simulink model "Khan_hw_3"  (R2021a)
settings: Solver=VariableStepAuto  StartTime=0.0  StopTime=10.0  RelTol=1e-3
values from neighbouring files (symbols this model uses):
  q0 = angle2quat(phidot,thetadot,psidot)    [khan_hw_3_script.m]
settings Model: Creator=ARK  LastModifiedBy=ARK

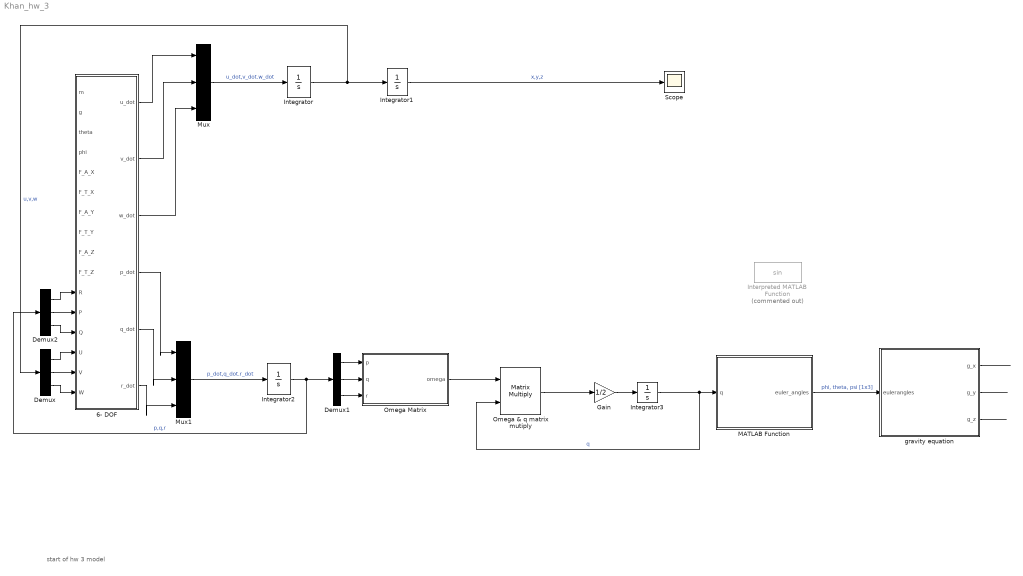
== system Khan_hw_3 ==
  note: start of hw 3 model
  6- DOF : MATLAB Function  TreatAsAtomicUnit=on
  Demux : Demux  Outputs=3
  Demux1 : Demux  Outputs=3
  Demux2 : Demux  Outputs=3
  Gain : Gain  Gain=1/2
  Integrator : Integrator  InitialCondition=1
  Integrator1 : Integrator  InitialCondition=1
  Integrator2 : Integrator  InitialCondition=1
  Integrator3 : Integrator  InitialCondition=q0
  Interpreted MATLAB Function : MATLABFcn  Commented=on
  MATLAB Function : MATLAB Function  TreatAsAtomicUnit=on
  Mux : Mux  Inputs=3
  Mux1 : Mux  Inputs=3
  Omega & q matrix mutiply : Product  Multiplication=Matrix(*)
  Omega Matrix : MATLAB Function  TreatAsAtomicUnit=on
  Scope : Scope
  gravity equation : MATLAB Function  TreatAsAtomicUnit=on
  wires:
  6- DOF/1(u_dot) -> Mux/1
  6- DOF/2(v_dot) -> Mux/2
  6- DOF/3(w_dot) -> Mux/3
  Mux/1 -> Integrator/1  "u_dot,v_dot.w_dot"
  Integrator/1 -> Integrator1/1, Demux/1  "u,v,w"
  Integrator1/1 -> Scope/1  "x,y,z"
  Demux/2 -> 6- DOF/15(V)
  Demux/1 -> 6- DOF/14(U)
  Demux/3 -> 6- DOF/16(W)
  6- DOF/4(p_dot) -> Mux1/1
  6- DOF/5(q_dot) -> Mux1/2
  6- DOF/6(r_dot) -> Mux1/3
  Mux1/1 -> Integrator2/1  "p_dot,q_dot.r_dot"
  Integrator2/1 -> Demux2/1, Demux1/1  "p,q,r"
  Demux1/1 -> Omega Matrix/1(p)
  Demux1/3 -> Omega Matrix/3(r)
  Demux1/2 -> Omega Matrix/2(q)
  Omega Matrix/1(omega) -> Omega & q matrix mutiply/1
  Omega & q matrix mutiply/1 -> Gain/1
  Gain/1 -> Integrator3/1
  Integrator3/1 -> Omega & q matrix mutiply/2, MATLAB Function/1(q)  "q"
  MATLAB Function/1(euler_angles) -> gravity equation/1(eulerangles)  "phi, theta, psi [1x3]"
  gravity equation/1(g_x) -> ?
  gravity equation/2(g_y) -> ?
  gravity equation/3(g_z) -> ?
  Demux2/1 -> 6- DOF/11(R)
  Demux2/2 -> 6- DOF/12(P)
  Demux2/3 -> 6- DOF/13(Q)

== matlab function Khan_hw_3/Omega Matrix ==
  data: p input; omega output; q input; r input
function omega = fcn(p,q,r)


wx = p;
wy = q;
wz = r;
omega = [0 -wx -wy -wz;
    wx 0 wz -wy;
    wy -wz 0 wx;
    wz wy -wx 0];

== matlab function Khan_hw_3/6- DOF ==
  data: m input; u_dot output; v_dot output; w_dot output; g input; theta input; phi input; F_A_X input; F_T_X input; F_A_Y input; F_T_Y input; F_A_Z input; F_T_Z input; R input; P input; Q input; U input; V input; W input; p_dot output; q_dot output; r_dot output



function [u_dot,v_dot,w_dot,p_dot,q_dot,r_dot] = fcn(m,g,theta,phi,F_A_X,F_T_X,F_A_Y,F_T_Y,F_A_Z,F_T_Z,R,P,Q,U,V,W)

% CLMEs
u_dot = (1/m)*(-m*g*sin(theta)+F_A_X+F_T_X)-(Q*W)+(R*V);
v_dot = (1/m)*(-m*g*sin(theta)+F_A_Y+F_T_Y)-(U*R)+(P*W);
w_dot = (1/m)*(-m*g*sin(theta)+F_A_Z+F_T_Z)-(P*V)+(Q*U);

%CAMEs
% [We are doing CAMEs. So KEs,GEs, and FPEs]
p_dot = (1/I_XX)*((r_dot*I_XZ)+(P*Q*I_XZ)-((R*Q)*(I_ZZ-I_YY))+L_A+L_T);
q_dot = (1/I_YY)*((-P*R*(I_XX-I_ZZ))-(I_XZ*(P^2-R^2))+M_A+M_T);
r_dot = (1/I_ZZ)*((p_dot*I_XZ)-(P*Q)*(I_YY-I_XX)-(Q*R*I_XZ)+N_A+N_T);

== matlab function Khan_hw_3/MATLAB Function ==
  data: q input; euler_angles output
function euler_angles = WrapperQuat2Angle(q)

[psi,theta,phi] = quat2angle(q');

euler_angles = [phi;theta;psi];
end

== matlab function Khan_hw_3/gravity equation ==
  data: eulerangles input; g_x output; g_y output; g_z output
function [g_x,g_y,g_z] = fcn(eulerangles)

g_x = -g*sin(eulerangles(2));
g_y = g*cos(eulerangles(2))*sin(eulerangles(1));
g_z = g*cos(eulerangles(2))*cos(eulerangles(1));
